simulink model "uav_sim"  (R2022b)
settings: Solver=VariableStepAuto  StartTime=0.0  StopTime=10  RelTol=1e-3
PreLoadFcn:
  | load('quad_params.mat')
values from neighbouring files (symbols this model uses):
  quad_m = [1.37953125e-07 9.75475901734e-09 9.75475901734e-09 3.12206222222e-09 1.37953125e-07 -9.75475901734e-09 9.75475901734e-09 -3.12206222222e-09 1.37953125e-07 -9.75475901734e-09 -9.75475901734e-09 3.12206222222e-09 ... (16 elements, 4x4)]    [quad_params.mat]
  W = 8.829    [quad_params.mat]
libraries: shared6dof x1, robotcorelib x1, sharedtransform x1, aerolibanimutils x1, uavutilslib x1
settings Model: Creator=Aorus PC  LastModifiedBy=Aorus PC

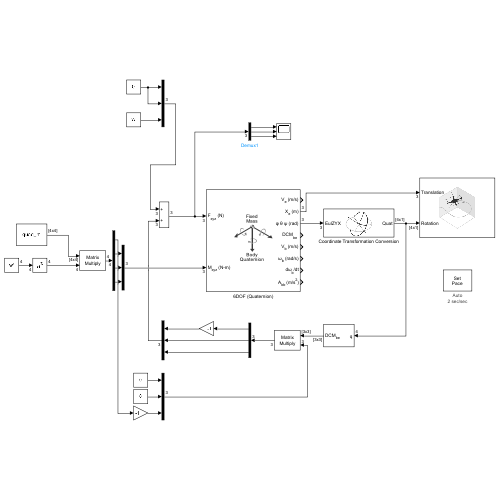
[thumbnail: Simulink's stored preview of the top-level diagram]
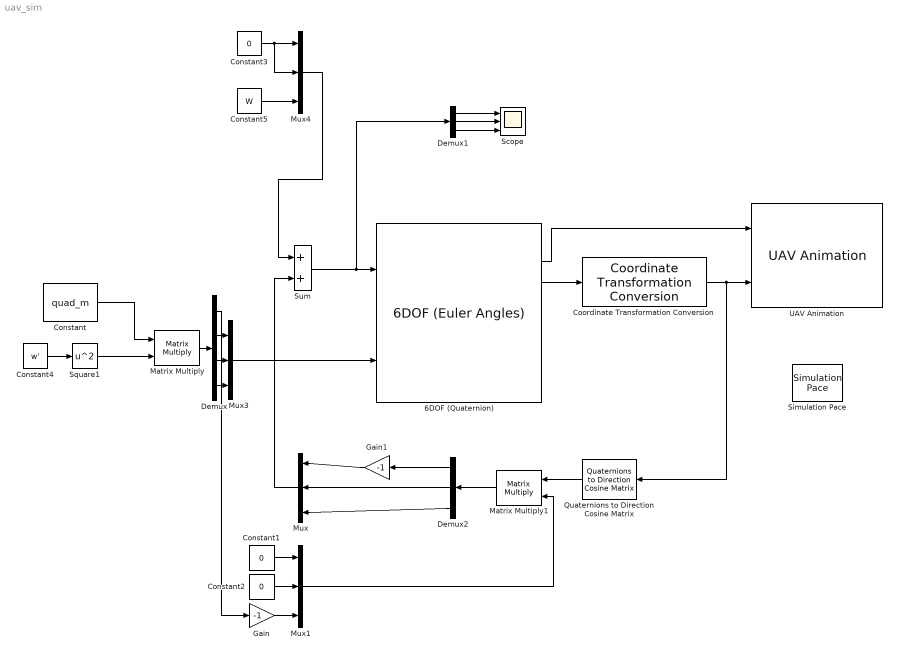
== system uav_sim ==
  6DOF (Quaternion) : shared6dof/6DOF (Euler Angles)  units=Metric (MKS)  mtype=Fixed  rep=Quaternion  xme_0=[0 0 0]  Vm_0=[0 0 0]  eul_0=[0 0 0]  pm_0=[0 0 0]  mass_0=1.0  mass_e=0.5  mass_f=2.0  inertia=eye(3)  inertia_e=eye(3)  inertia_f=2*eye(3)  k_quat=1.0  vre_flag=on  abi_flag=off  aMode=0  xme_statename=''  Vm_statename=''  eul_statename=''  quat_statename=''  pm_statename=''  mass_statename=''
      settings: LibrarySourceBlock=aerolib6dof2/6DOF (Quaternion)
  Constant : Constant  Value=quad_m
  Constant1 : Constant  Value=0
  Constant2 : Constant  Value=0
  Constant3 : Constant  Value=0
  Constant4 : Constant  Value=w'
  Constant5 : Constant  Value=W
  Coordinate Transformation Conversion : robotcorelib/Coordinate Transformation Conversion  InputRepresentation=Euler Angles  InputEulerSequence=ZYX  ShowTrVecInputPort=on  OutputRepresentation=Quaternion  OutputEulerSequence=ZYX  ShowTrVecOutputPort=on  SimulateUsing=Interpreted execution
      settings: LibrarySourceBlock=uavutilslib/Coordinate Transformation Conversion
  Demux : Demux
  Demux1 : Demux  Outputs=3
  Demux2 : Demux  Outputs=3
  Gain : Gain  Gain=-1
  Gain1 : Gain  Gain=-1
  Matrix Multiply : Product  Multiplication=Matrix(*)
  Matrix Multiply1 : Product  Multiplication=Matrix(*)
  Mux{,1,3..4} (4 alike) : Mux  Inputs=3
  Quaternions to Direction Cosine Matrix : sharedtransform/Quaternions to  Direction Cosine Matrix  aMode=aMode
      settings: LibrarySourceBlock=|
      | aerolibtransform2/Quaternions to
      | Direction Cosine Matrix
  Scope : Scope  NumInputPorts=3
  Simulation Pace : aerolibanimutils/Simulation Pace  SimulationPace=2  SleepMode=Auto  OutputPaceError=off  SampleTime=1/30
  Square1 : Math  Operator=square
  Sum : Sum
  UAV Animation : uavutilslib/UAV Animation  UAVType=Multirotor  UAVSize=4  InertialZDirection=Down  SampleTime=-1
  wires:
  Coordinate Transformation Conversion/1 -> Quaternions to Direction Cosine Matrix/1, UAV Animation/2
  6DOF (Quaternion)/2 -> UAV Animation/1
  Constant/1 -> Matrix Multiply/1
  6DOF (Quaternion)/3 -> Coordinate Transformation Conversion/1
  Matrix Multiply/1 -> Demux/1
  Demux/2 -> Mux3/1
  Demux/3 -> Mux3/2
  Demux/4 -> Mux3/3
  Mux3/1 -> 6DOF (Quaternion)/2
  Constant3/1 -> Mux4/2, Mux4/1
  Constant5/1 -> Mux4/3
  Mux4/1 -> Sum/1
  Constant2/1 -> Mux1/2
  Constant1/1 -> Mux1/1
  Square1/1 -> Matrix Multiply/2
  Demux/1 -> Gain/1
  Gain/1 -> Mux1/3
  Constant4/1 -> Square1/1
  Quaternions to Direction Cosine Matrix/1 -> Matrix Multiply1/1
  Mux1/1 -> Matrix Multiply1/2
  Mux/1 -> Sum/2
  Demux1/2 -> Scope/2
  Demux1/1 -> Scope/1
  Demux1/3 -> Scope/3
  Sum/1 -> 6DOF (Quaternion)/1, Demux1/1
  Demux2/1 -> Gain1/1
  Demux2/3 -> Mux/3
  Matrix Multiply1/1 -> Demux2/1
  Gain1/1 -> Mux/1
  Demux2/2 -> Mux/2
